simulink model "fig2_8"  (R2026a)
settings: Solver=ode15s  StopTime=50  MaxStep=0.005  RelTol=1e-6  AbsTol=1e-8
values from neighbouring files (symbols this model uses):
  qco = 1.1    [Comparisons_of_Examples_OLOP_Jump_Frequency.m]    (also in OLOP_GUI.m = qcoEdit.Value; gilbreathDF_v3.m; gilbreathJumpPhenomena.m; jump_phenomena_soft_glide.m)
  R = 15    [Comparisons_of_Examples_OLOP_Jump_Frequency.m]    (also in Fig16_OLOP_Nichols.m = 5; LimitCycleAnalysisbyNIDF_GUI.m = appData.R.Value; OLOP_GUI.m = REdit.Value; Olop_nichols_fig16.m = 5)
  w = logspace(-1, 2, n)    [Comparisons_of_Examples_OLOP_Jump_Frequency.m]    (also in Fig16_OLOP_Nichols.m = sort(unique([w_log, w_dens])); OLOP_GUI.m; Olop_nichols_fig16.m = logspace(log10(w_onset/100), log10(w_onset*100), 1200); aircraft_limit_cycle_describing_function.m = logspace(-3, 3, 30000))
settings Model: Creator=t0900  LastModifiedBy=t0900

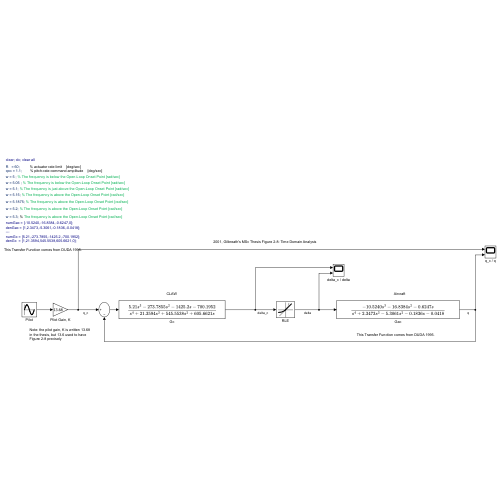
[thumbnail: Simulink's stored preview of the top-level diagram]
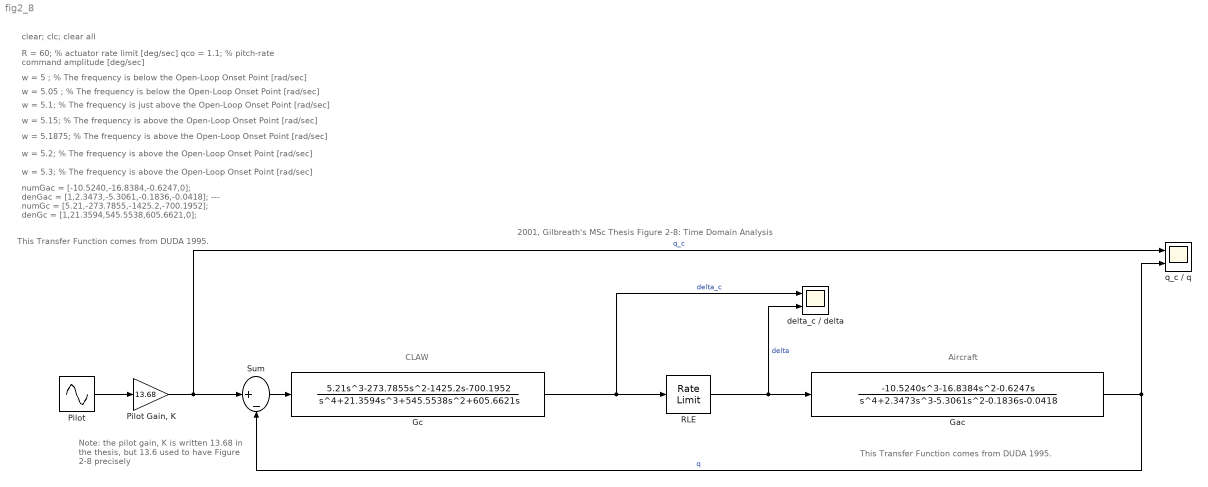
== system fig2_8 ==
  note: This Transfer Function comes from DUDA 1995.
  note: Note: the pilot gain, K is written 13.68 in the thesis, but 13.6 used to have Figure 2-8 precisely
  note: 2001, Gilbreath's MSc Thesis Figure 2-8: Time Domain Analysis
  note: CLAW
  note: Aircraft
  note: numGac = [-10.5240,-16.8384,-0.6247,0];
      | denGac = [1,2.3473,-5.3061,-0.1836,-0.0418];
      | ---
      | numGc = [5.21,-273.7855,-1425.2,-700.1952];
      | denGc  = [1,21.3594,545.5538,605.6621,0];
  note: R = 60; % actuator rate limit [deg/sec]
      | qco = 1.1; % pitch-rate command amplitude [deg/sec]
  note: clear; clc; clear all
  note: w = 5.3; % The frequency is above the Open-Loop Onset Point [rad/sec]
  note: w = 5 ; % The frequency is below the Open-Loop Onset Point [rad/sec]
  note: w = 5.1; % The frequency is just above the Open-Loop Onset Point [rad/sec]
  note: w = 5.2; % The frequency is above the Open-Loop Onset Point [rad/sec]
  note: w = 5.05 ; % The frequency is below the Open-Loop Onset Point [rad/sec]
  note: w = 5.15; % The frequency is above the Open-Loop Onset Point [rad/sec]
  note: w = 5.1875; % The frequency is above the Open-Loop Onset Point [rad/sec]
  note: This Transfer Function comes from DUDA 1995.
  Gac : TransferFcn  Numerator=[-10.5240, -16.8384 ,-0.6247, 0]  Denominator=[1,2.3473,-5.3061,-0.1836,-0.0418]
  Gc : TransferFcn  Numerator=[5.21,-273.7855,-1425.2,-700.1952]  Denominator=[1,21.3594,545.5538,605.6621,0]
  Pilot : Sin  Amplitude=qco  Frequency=w  SampleTime=0
  "Pilot Gain, K" : Gain  Gain=13.68
  RLE : RateLimiter  RisingSlewLimit=R  FallingSlewLimit=-R
  Sum : Sum  Inputs=|+-
  delta_c / delta : Scope  NumInputPorts=2
      settings: ActiveDisplayYMinimum=10.528938257550703  ActiveDisplayYMaximum=15.190309448178303  YLabel=degrees
  q_c / q : Scope  NumInputPorts=2
      settings: ActiveDisplayYMinimum=-43.294515420005212  ActiveDisplayYMaximum=40.857407707522412  YLabel=deg/sec  DataLoggingVariableName=ScopeData2
  wires:
  Pilot/1 -> "Pilot Gain, K"/1
  "Pilot Gain, K"/1 -> q_c / q/1, Sum/1  "q_c"
  Sum/1 -> Gc/1
  Gc/1 -> delta_c / delta/1, RLE/1  "delta_c"
  RLE/1 -> Gac/1, delta_c / delta/2  "delta"
  Gac/1 -> q_c / q/2, Sum/2  "q"
